simulink model "VOO"  (R2023a)
settings: Solver=FixedStepAuto  StartTime=0.0  StopTime=10.0  FixedStep=1e-3  RelTol=1e-3  EnableMultiTasking=on
settings Model: ExtModeTrigDuration=5  Creator=tstic  LastModifiedBy=avala
settings OptimizationCC: EnhancedBackFolding=on  PassReuseOutputArgsAs=Individual arguments  ZeroExternalMemoryAtStartup=off  ZeroInternalMemoryAtStartup=off  MaxStackSize=64  OptimizeBlockOrder=speed  DifferentSizesBufferReuse=on  OptimizationCustomize=off  EfficientTunableParamExpr=on
settings DebuggingCC: ParameterTunabilityLossMsg=error
settings HardwareCC: ProdBitPerPointer=32  ProdBitPerSizeT=32  ProdBitPerPtrDiffT=32  ProdLargestAtomicInteger=Long  ProdLargestAtomicFloat=Double  ProdWordSize=32  ProdHWDeviceType=ARM Compatible->ARM Cortex
settings SFSimCC: MATLABDynamicMemAlloc=off
settings RTWCC: Description=Embedded Coder  SystemTargetFile=ert.tlc  HardwareBoard=NXP FRDM-K64F  TLCOptions="-aInlineSetEventsForThisBaseRateFcn=TLC_FALSE -aSuppressMultiTaskScheduler=TLC_FALSE  -aRateBasedStepFcn=0"  TemplateMakefile=ert_default_tmf  Toolchain=GNU Tools for ARM Embedded Processors
settings CodeAppCC: ForceParamTrailComments=on  IgnoreCustomStorageClasses=off  OperatorAnnotations=on  SimulinkDataObjDesc=on  SFDataObjDesc=on  InsertBlockDesc=on
settings ERTTargetCC: ExtModeTransport=4  ExtModeMexFile=sendToCommService

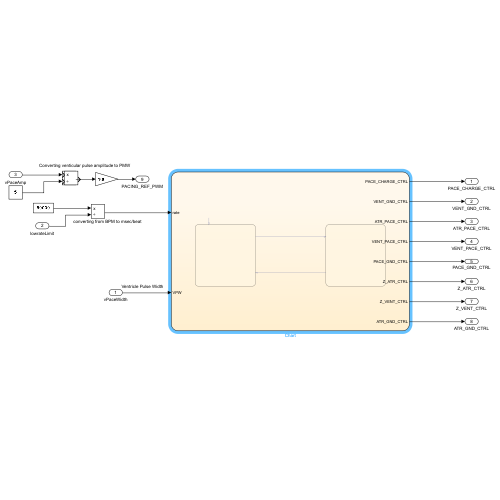
[thumbnail: Simulink's stored preview of the top-level diagram]
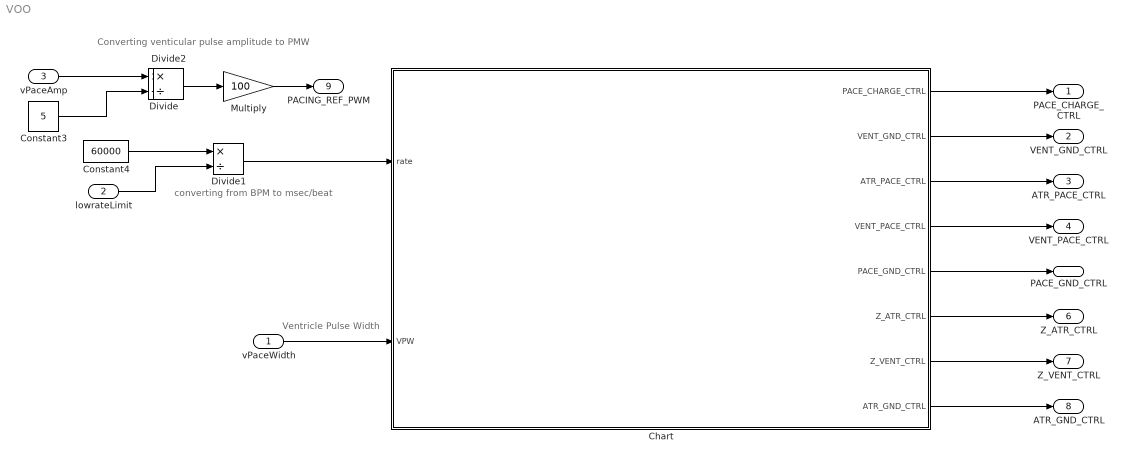
== system VOO ==
  note: Converting venticular pulse amplitude to PMW
  note: Ventricle Pulse Width
  note: converting from BPM to msec/beat
  vPaceWidth : Inport
  lowrateLimit : Inport  Port=2
  vPaceAmp : Inport  Port=3
  Chart : Stateflow chart  TreatAsAtomicUnit=on
  Constant3 : Constant  Value=5
  Constant4 : Constant  Value=60000
  Divide : Product  Inputs=*/
  Divide1 : Product  Inputs=*/
  Divide2 : Product  Inputs=*/
  Multiply : Gain  Gain=100
  PACE_CHARGE_CTRL : Outport
  VENT_GND_CTRL : Outport  Port=2
  ATR_PACE_CTRL : Outport  Port=3
  VENT_PACE_CTRL : Outport  Port=4
  PACE_GND_CTRL : Outport  Port=5
  Z_ATR_CTRL : Outport  Port=6
  Z_VENT_CTRL : Outport  Port=7
  ATR_GND_CTRL : Outport  Port=8
  PACING_REF_PWM : Outport  Port=9
  wires:
  Chart/1(PACE_CHARGE_CTRL) -> PACE_CHARGE_CTRL/1
  Chart/2(VENT_GND_CTRL) -> VENT_GND_CTRL/1
  vPaceWidth/1 -> Chart/2(VPW)
  Divide1/1 -> Chart/1(rate)
  Chart/3(ATR_PACE_CTRL) -> ATR_PACE_CTRL/1
  Chart/4(VENT_PACE_CTRL) -> VENT_PACE_CTRL/1
  Chart/5(PACE_GND_CTRL) -> PACE_GND_CTRL/1
  Chart/6(Z_ATR_CTRL) -> Z_ATR_CTRL/1
  Chart/7(Z_VENT_CTRL) -> Z_VENT_CTRL/1
  Chart/8(ATR_GND_CTRL) -> ATR_GND_CTRL/1
  Constant3/1 -> Divide/2
  Divide/1 -> Multiply/1
  vPaceAmp/1 -> Divide/1
  Multiply/1 -> PACING_REF_PWM/1
  lowrateLimit/1 -> Divide1/2
  Constant4/1 -> Divide1/1

== stateflow chart VOO/Chart ==
  state Charging
    %charges and discharges
    entry:
    PACE_GND_CTRL = 1;
    VENT_PACE_CTRL = 0;
    Z_ATR_CTRL = 0;
    Z_VENT_CTRL = 0;
    ATR_PACE_CTRL = 0;
    ATR_GND_CTRL = 0;
    VENT_GND_CTRL = 1;
    during:
    PACE_CHARGE_CTRL = 1;
  state Pacing_Ventricle
    %pacing
    entry:
    PACE_CHARGE_CTRL = 0;
    PACE_GND_CTRL = 1;
    ATR_PACE_CTRL = 0;
    ATR_GND_CTRL = 0;
    Z_ATR_CTRL = 0;
    Z_VENT_CTRL = 0;
    VENT_GND_CTRL = 0;
    VENT_PACE_CTRL = 1;
  note: Pacing ventricle at rate of lowrateLimit
  note: Pacing ventricle for duration of ventricle pulse width
  (default) -> Charging
  Charging -> Pacing_Ventricle : after(rate-VPW,msec)
  Pacing_Ventricle -> Charging : after(VPW,msec)
  data: PACE_CHARGE_CTRL output; VENT_GND_CTRL output; ATR_PACE_CTRL output; VENT_PACE_CTRL output; PACE_GND_CTRL output; Z_ATR_CTRL output; Z_VENT_CTRL output; rate input; ATR_GND_CTRL output; VPW input
